simulink model "simulation_TF"  (R2023b)
settings: Solver=VariableStepAuto  StartTime=0.0  StopTime=100  RelTol=1e-3
libraries: SignalEditorBlockLib x3
settings Model: Creator=David  LastModifiedBy=David
settings RTWCC: GPUComputeCapability=5.0
settings ConfigComp: CovBoundaryAbsTol=1.0e-5

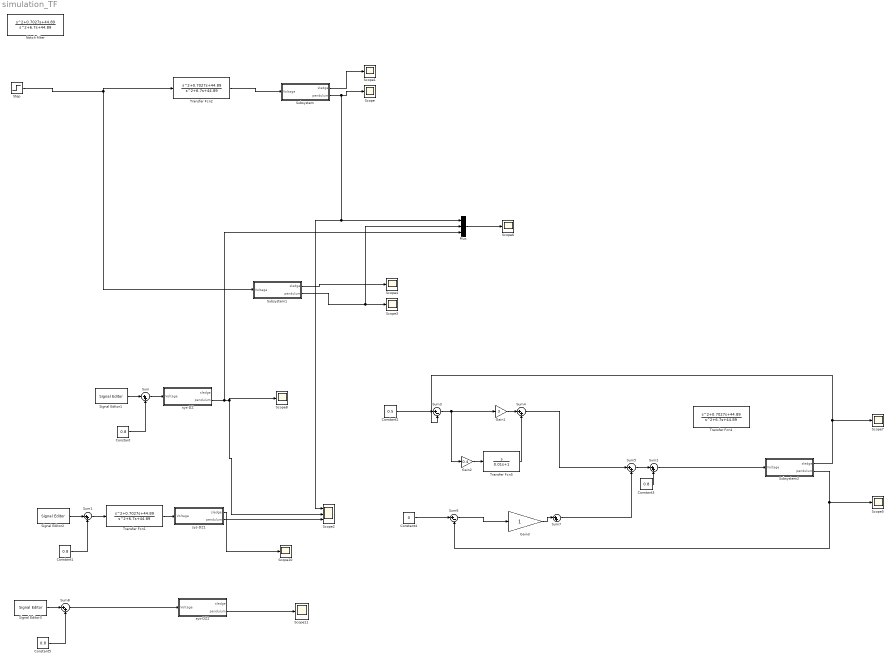
== system simulation_TF ==
  Constant{,1,3,5} (4 alike) : Constant  Value=0.8
  Constant2 : Constant  Value=0.5
  Constant4 : Constant  Value=0
  Gain1 : Gain  Gain=3
  Gain2 : Gain  Gain=0.4
  Gain3 : Gain
  Mux : Mux  Inputs=3
  "Notch filter " : TransferFcn  Numerator=[1 0.7027 44.89]  Denominator=[1 6.7 44.89]
  Scope{,1,3..8,10..11} (10 alike) : Scope
  Scope2 : Scope  NumInputPorts=3
  Signal Editor1 : SignalEditorBlockLib/Signal Editor  FileName=signal_input2.mat  ActiveScenario=Scenario  ActiveSignal=Signal 1  IsBus=off  OutputBusObjectStr=Bus: BusObject  SampleTime=0  ZeroCross=off  OutputAfterFinalValue=Setting to zero  Unit=inherit  PreserveSignalName=on  ApplySigPropsToAllScenarios=on  ApplySigPropsToAllSignals=off
  Signal Editor2 : SignalEditorBlockLib/Signal Editor  FileName=signal_input2.mat  ActiveScenario=Scenario  ActiveSignal=Signal 1  IsBus=off  OutputBusObjectStr=Bus: BusObject  SampleTime=0  ZeroCross=off  OutputAfterFinalValue=Setting to zero  Unit=inherit  PreserveSignalName=on  ApplySigPropsToAllScenarios=on  ApplySigPropsToAllSignals=off
  Signal Editor3 : SignalEditorBlockLib/Signal Editor  FileName=signal_input2.mat  ActiveScenario=Scenario  ActiveSignal=Signal 1  IsBus=off  OutputBusObjectStr=Bus: BusObject  SampleTime=0  ZeroCross=off  OutputAfterFinalValue=Setting to zero  Unit=inherit  PreserveSignalName=on  ApplySigPropsToAllScenarios=on  ApplySigPropsToAllSignals=off
  Step : Step  Time=2  Before=1.3  After=0  SampleTime=0
  Subsystem : Subsystem
  Subsystem1 : Subsystem
  Subsystem2 : Subsystem
  Sum{,1..2,4..5,7..8} (7 alike) : Sum  Inputs=|++
  Sum3 : Sum  Inputs=|+-
  Sum6 : Sum  Inputs=|+-
  Transfer Fcn1 : TransferFcn  Numerator=[1 0.7027 44.89]  Denominator=[1 6.7 44.89]
  Transfer Fcn2 : TransferFcn  Numerator=[1 0.7027 44.89]  Denominator=[1 6.7 44.89]
  Transfer Fcn4 : TransferFcn  Numerator=[1 0.7027 44.89]  Denominator=[1 6.7 44.89]
  Transfer Fcn5 : TransferFcn  Numerator=[1 0]  Denominator=[0.01 1]
  sys-DZ : Subsystem
  sys-DZ1 : Subsystem
  sys-DZ2 : Subsystem
  wires:
  Step/1 -> Subsystem1/1(Voltage), Transfer Fcn2/1
  Subsystem/2(pendulum) -> Mux/1, Scope2/1, Scope/1
  Subsystem/1(sledge) -> Scope1/1
  Subsystem1/1(sledge) -> Scope4/1
  Subsystem1/2(pendulum) -> Mux/2, Scope3/1
  Transfer Fcn2/1 -> Subsystem/1(Voltage)
  Mux/1 -> Scope6/1
  Signal Editor1/1 -> Sum/1
  sys-DZ/2(pendulum) -> Mux/3, Scope2/2, Scope8/1
  Sum/1 -> sys-DZ/1(Voltage)
  Constant/1 -> Sum/2
  Constant1/1 -> Sum1/2
  Sum1/1 -> Transfer Fcn1/1
  Signal Editor2/1 -> Sum1/1
  Transfer Fcn1/1 -> sys-DZ1/1(Voltage)
  sys-DZ1/2(pendulum) -> Scope2/3
  Gain1/1 -> Sum4/1
  Subsystem2/2(pendulum) -> Scope5/1, Sum6/2
  Constant2/1 -> Sum3/1
  Subsystem2/1(sledge) -> Sum3/2, Scope7/1
  Constant3/1 -> Sum2/2
  Sum2/1 -> Subsystem2/1(Voltage)
  sys-DZ1/1(sledge) -> Scope10/1
  Sum4/1 -> Sum5/1
  Sum5/1 -> Sum2/1
  Sum7/1 -> Sum5/2
  Gain3/1 -> Sum7/1
  Constant4/1 -> Sum6/1
  Sum6/1 -> Gain3/1
  Sum3/1 -> Gain2/1, Gain1/1
  Gain2/1 -> Transfer Fcn5/1
  Transfer Fcn5/1 -> Sum4/2
  Signal Editor3/1 -> Sum8/1
  Constant5/1 -> Sum8/2
  Sum8/1 -> sys-DZ2/1(Voltage)
  sys-DZ2/2(pendulum) -> Scope11/1

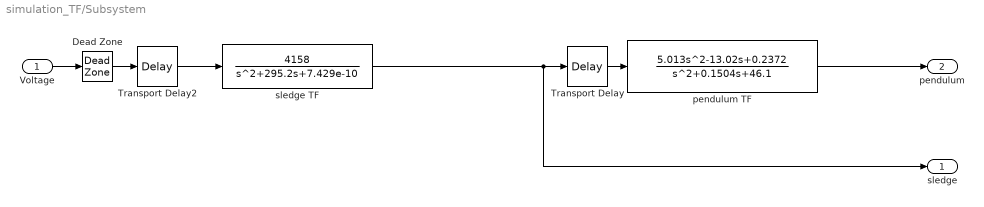
== system simulation_TF/Subsystem ==
  Voltage : Inport
  Dead Zone : DeadZone  LowerValue=-0.8  UpperValue=0.8
  Transport Delay : TransportDelay  DelayTime=0.07
  Transport Delay2 : TransportDelay  DelayTime=0.02
  pendulum TF : TransferFcn  Numerator=[5.013 -13.02 0.2372]  Denominator=[1 0.1504 46.1]
  sledge TF : TransferFcn  Numerator=[4158]  Denominator=[1 295.2 7.429e-10]
  sledge : Outport
  pendulum : Outport  Port=2
  wires:
  pendulum TF/1 -> pendulum/1
  Voltage/1 -> Dead Zone/1
  sledge TF/1 -> sledge/1, Transport Delay/1
  Transport Delay/1 -> pendulum TF/1
  Dead Zone/1 -> Transport Delay2/1
  Transport Delay2/1 -> sledge TF/1

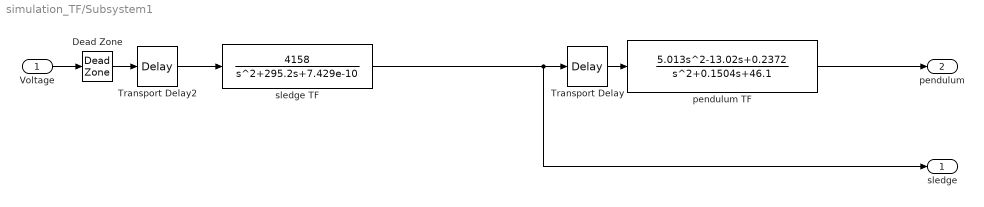
== system simulation_TF/Subsystem1 ==
  Voltage : Inport
  Dead Zone : DeadZone  LowerValue=-0.8  UpperValue=0.8
  Transport Delay : TransportDelay  DelayTime=0.07
  Transport Delay2 : TransportDelay  DelayTime=0.02
  pendulum TF : TransferFcn  Numerator=[5.013 -13.02 0.2372]  Denominator=[1 0.1504 46.1]
  sledge TF : TransferFcn  Numerator=[4158]  Denominator=[1 295.2 7.429e-10]
  sledge : Outport
  pendulum : Outport  Port=2
  wires:
  Transport Delay2/1 -> sledge TF/1
  Dead Zone/1 -> Transport Delay2/1
  Transport Delay/1 -> pendulum TF/1
  sledge TF/1 -> Transport Delay/1, sledge/1
  Voltage/1 -> Dead Zone/1
  pendulum TF/1 -> pendulum/1

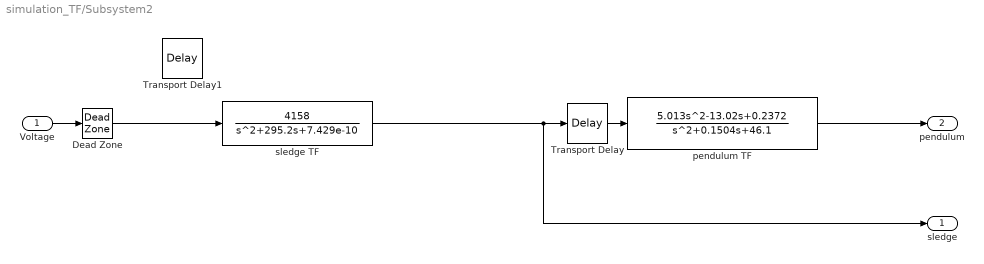
== system simulation_TF/Subsystem2 ==
  Voltage : Inport
  Dead Zone : DeadZone  LowerValue=-0.8  UpperValue=0.8
  Transport Delay : TransportDelay  DelayTime=0.07
  Transport Delay1 : TransportDelay  DelayTime=0.02
  pendulum TF : TransferFcn  Numerator=[5.013 -13.02 0.2372]  Denominator=[1 0.1504 46.1]
  sledge TF : TransferFcn  Numerator=[4158]  Denominator=[1 295.2 7.429e-10]
  sledge : Outport
  pendulum : Outport  Port=2
  wires:
  Dead Zone/1 -> sledge TF/1
  Transport Delay/1 -> pendulum TF/1
  sledge TF/1 -> Transport Delay/1, sledge/1
  Voltage/1 -> Dead Zone/1
  pendulum TF/1 -> pendulum/1

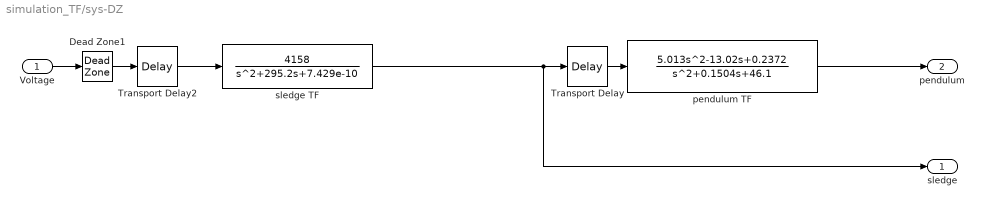
== system simulation_TF/sys-DZ ==
  Voltage : Inport
  Dead Zone1 : DeadZone  LowerValue=-0.8  UpperValue=0.8
  Transport Delay : TransportDelay  DelayTime=0.07
  Transport Delay2 : TransportDelay  DelayTime=0.02
  pendulum TF : TransferFcn  Numerator=[5.013 -13.02 0.2372]  Denominator=[1 0.1504 46.1]
  sledge TF : TransferFcn  Numerator=[4158]  Denominator=[1 295.2 7.429e-10]
  sledge : Outport
  pendulum : Outport  Port=2
  wires:
  Transport Delay2/1 -> sledge TF/1
  Voltage/1 -> Dead Zone1/1
  Transport Delay/1 -> pendulum TF/1
  sledge TF/1 -> Transport Delay/1, sledge/1
  pendulum TF/1 -> pendulum/1
  Dead Zone1/1 -> Transport Delay2/1

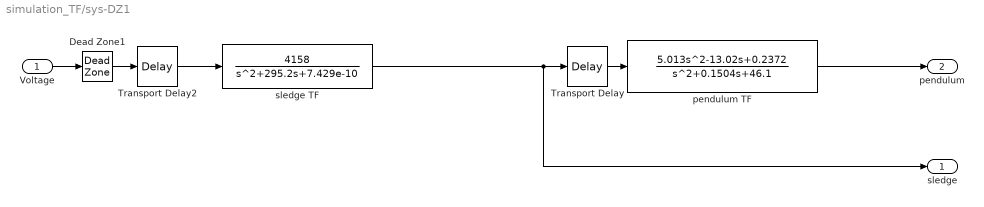
== system simulation_TF/sys-DZ1 ==
  Voltage : Inport
  Dead Zone1 : DeadZone  LowerValue=-0.8  UpperValue=0.8
  Transport Delay : TransportDelay  DelayTime=0.07
  Transport Delay2 : TransportDelay  DelayTime=0.02
  pendulum TF : TransferFcn  Numerator=[5.013 -13.02 0.2372]  Denominator=[1 0.1504 46.1]
  sledge TF : TransferFcn  Numerator=[4158]  Denominator=[1 295.2 7.429e-10]
  sledge : Outport
  pendulum : Outport  Port=2
  wires:
  Transport Delay2/1 -> sledge TF/1
  Voltage/1 -> Dead Zone1/1
  Transport Delay/1 -> pendulum TF/1
  sledge TF/1 -> Transport Delay/1, sledge/1
  pendulum TF/1 -> pendulum/1
  Dead Zone1/1 -> Transport Delay2/1

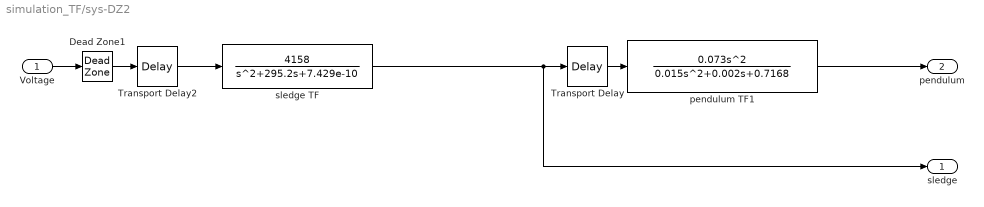
== system simulation_TF/sys-DZ2 ==
  Voltage : Inport
  Dead Zone1 : DeadZone  LowerValue=-0.8  UpperValue=0.8
  Transport Delay : TransportDelay  DelayTime=0.07
  Transport Delay2 : TransportDelay  DelayTime=0.02
  pendulum TF1 : TransferFcn  Numerator=[0.073 0 0]  Denominator=[0.015 0.002 0.7168]
  sledge TF : TransferFcn  Numerator=[4158]  Denominator=[1 295.2 7.429e-10]
  sledge : Outport
  pendulum : Outport  Port=2
  wires:
  Dead Zone1/1 -> Transport Delay2/1
  pendulum TF1/1 -> pendulum/1
  sledge TF/1 -> sledge/1, Transport Delay/1
  Transport Delay/1 -> pendulum TF1/1
  Voltage/1 -> Dead Zone1/1
  Transport Delay2/1 -> sledge TF/1
